simulink model "DC_motor_Fuzzy_pid_V3"  (R2020a)
settings: Solver=FixedStepAuto  StartTime=0.0  StopTime=7.5  FixedStep=0.001  RelTol=1e-3
undefined symbols (not defined in the file): sigbuilder_block
libraries: fuzblock x1
settings Model: Creator=kesha  LastModifiedBy=OMEN
settings DataIOCC: ReturnWorkspaceOutputs=off
settings DebuggingCC: ArithmeticOperatorsInVariantConditions=warning
settings SFSimCC: SimUseLocalCustomCode=off  CustomCodeUndefinedFunction=UseInterfaceOnly
settings RTWCC: RTWUseLocalCustomCode=off

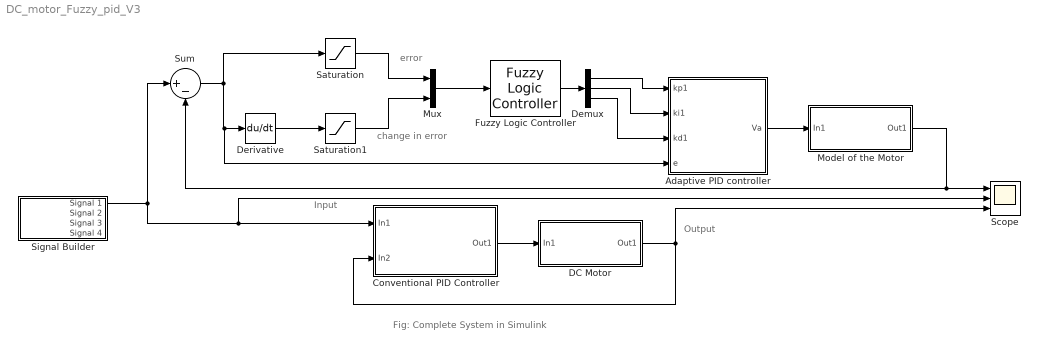
== system DC_motor_Fuzzy_pid_V3 ==
  note: change in error
  note: error
  note: Output
  note: Input
  note: Fig: Complete System in Simulink
  " Adaptive PID controller" : Subsystem  mask{Kp1=0.9989, Ki1=13.57, Kd1=0.01035}
      mask prompts: Kp1 "P"; Ki1 "I"; Kd1 "D"
      mask DialogControl ParameterGroupVar Prompt: Preliminary PID Gains
  Conventional PID Controller : Subsystem  mask{Kp=0.1, Ki=10, Kd=0.01}
      mask prompts: Kp "P"; Ki "I"; Kd "D"
  DC Motor : Subsystem
  Demux : Demux  Outputs=3
  Derivative : Derivative
  Fuzzy Logic Controller : fuzblock/Fuzzy Logic  Controller  FIS='fuzzypid.fis'  OutputSampleNumber=101  DataType=double  FuzzifiedInputs=off  RuleFiringStrengths=off  RuleOutputs=off  AggregatedOutputs=off  SimulateUsing=Interpreted execution  OutOfRangeInputValueMessage=warning  NoRuleFiredMessage=warning  EmptyOutputFuzzySetMessage=warning
  Model of the Motor : Subsystem
  Mux : Mux  Inputs=2
  Saturation : Saturate  UpperLimit=1  LowerLimit=-1  LinearizeAsGain=off  ZeroCross=off
  Saturation1 : Saturate  UpperLimit=1  LowerLimit=-1  LinearizeAsGain=off
  Scope : Scope  NumInputPorts=3
  Signal Builder : Subsystem  Tag=STV Subsys  LoadFcn=sigbuilder_block('load');  StartFcn=sigbuilder_block('start');  StopFcn=sigbuilder_block('stop');  ClipboardFcn=sigbuilder_block('clipboard');  mask(Sigbuilder block){tuvar=[0:10]}
      mask help: Simulink:masks:SigbuilderBlock_MD
      mask init:
      | if ~strcmp(get_param(bdroot(gcbh),'SimulationStatus'),'stopped') tuvar = sigbuilder_block('maskInit'); end
      settings: CopyFcn=sigbuilder_block('copy');  DeleteFcn=sigbuilder_block('delete');  ModelCloseFcn=sigbuilder_block('modelClose');  PreSaveFcn=sigbuilder_block('preSave');  PauseFcn=sigbuilder_block('pause');  ContinueFcn=sigbuilder_block('continue');  NameChangeFcn=sigbuilder_block('namechange');  OpenFcn=sigbuilder_block('open',[148.8 141 550.8 400.2 ]);  CloseFcn=sigbuilder_block('close');
      mask Display: plot(0, 0, 100, 100,[2, 2, 32, 32, 2], [68, 8, 8, 68, 68],[32, 2], [38, 38], [32, 19, 2],[53, 60, 44], [32, 17, 17, 2],[16, 16, 31, 31]);txt = getActiveGroup(gcbh);text(2, 100, txt,'verticalAlignment', 'top');
  Sum : Sum  Inputs=|+-
  wires:
  Model of the Motor/1(Out1) -> Scope/1, Sum/2
  " Adaptive PID controller"/1(Va) -> Model of the Motor/1(In1)
  Sum/1 -> Saturation/1, " Adaptive PID controller"/4(e), Derivative/1
  Derivative/1 -> Saturation1/1
  Saturation/1 -> Mux/1
  Saturation1/1 -> Mux/2
  Fuzzy Logic Controller/1 -> Demux/1
  Demux/1 -> " Adaptive PID controller"/1(kp1)
  Demux/2 -> " Adaptive PID controller"/2(ki1)
  Demux/3 -> " Adaptive PID controller"/3("kd1 ")
  Signal Builder/1(Signal 1) -> Scope/2, Conventional PID Controller/1(In1), Sum/1
  DC Motor/1(Out1) -> Scope/3, Conventional PID Controller/2(In2)
  Mux/1 -> Fuzzy Logic Controller/1
  Conventional PID Controller/1(Out1) -> DC Motor/1(In1)

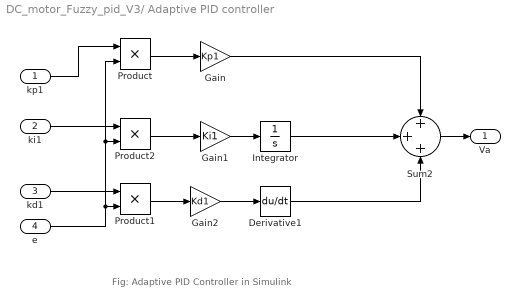
== system DC_motor_Fuzzy_pid_V3/ Adaptive PID controller ==
  note: Fig: Adaptive PID Controller in Simulink
  kp1 : Inport
  ki1 : Inport  Port=2
  "kd1 " : Inport  Port=3
  e : Inport  Port=4
  Derivative1 : Derivative
  Gain : Gain  Gain=Kp1
  Gain1 : Gain  Gain=Ki1
  Gain2 : Gain  Gain=Kd1
  Integrator : Integrator
  Product : Product
  Product1 : Product
  Product2 : Product
  Sum2 : Sum  Inputs=+++
  Va : Outport  VectorParamsAs1DForOutWhenUnconnected=off
  wires:
  Gain2/1 -> Derivative1/1
  Gain1/1 -> Integrator/1
  Sum2/1 -> Va/1
  kp1/1 -> Product/1
  ki1/1 -> Product2/1
  "kd1 "/1 -> Product1/1
  e/1 -> Product/2, Product2/2, Product1/2
  Gain/1 -> Sum2/1
  Integrator/1 -> Sum2/2
  Derivative1/1 -> Sum2/3
  Product/1 -> Gain/1
  Product2/1 -> Gain1/1
  Product1/1 -> Gain2/1

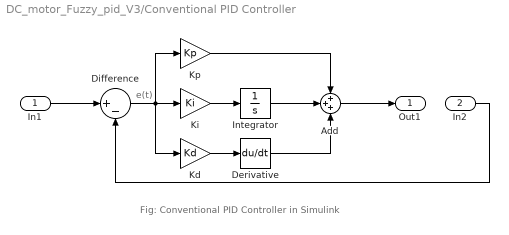
== system DC_motor_Fuzzy_pid_V3/Conventional PID Controller ==
  note: e(t)
  note: Fig: Conventional PID Controller in Simulink
  In1 : Inport
  In2 : Inport  Port=2
  " Derivative" : Derivative
  Add : Sum  Inputs=+++
  Difference : Sum  Inputs=|+-
  Integrator : Integrator
  Kd : Gain  Gain=Kd
  Ki : Gain  Gain=Ki
  Kp : Gain  Gain=Kp
  Out1 : Outport  VectorParamsAs1DForOutWhenUnconnected=off
  wires:
  " Derivative"/1 -> Add/3
  Ki/1 -> Integrator/1
  In2/1 -> Difference/2
  Integrator/1 -> Add/2
  Add/1 -> Out1/1
  In1/1 -> Difference/1
  Difference/1 -> Kd/1, Ki/1, Kp/1
  Kp/1 -> Add/1
  Kd/1 -> " Derivative"/1

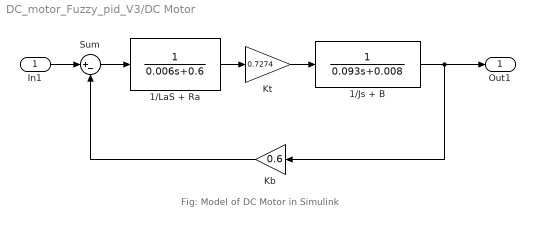
== system DC_motor_Fuzzy_pid_V3/DC Motor ==
  note: Fig: Model of DC Motor in Simulink
  In1 : Inport
  1/Js + B : TransferFcn  Denominator=[0.093 0.008]
  1/LaS + Ra : TransferFcn  Denominator=[0.006 0.6]
  Kb : Gain  Gain=0.6
  Kt : Gain  Gain=0.7274
  Sum : Sum  Inputs=|+-
  Out1 : Outport  VectorParamsAs1DForOutWhenUnconnected=off
  wires:
  1/LaS + Ra/1 -> Kt/1
  1/Js + B/1 -> Out1/1, Kb/1
  Kt/1 -> 1/Js + B/1
  Kb/1 -> Sum/2
  In1/1 -> Sum/1
  Sum/1 -> 1/LaS + Ra/1

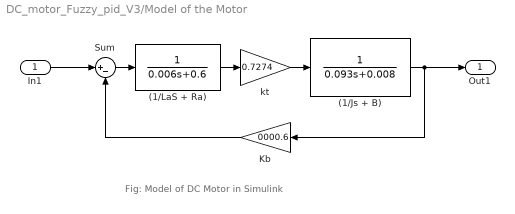
== system DC_motor_Fuzzy_pid_V3/Model of the Motor ==
  note: Fig: Model of DC Motor in Simulink
  In1 : Inport
  (1/Js + B) : TransferFcn  Denominator=[0.093 0.008]
  (1/LaS + Ra) : TransferFcn  Denominator=[0.006 0.6]
  Kb : Gain  Gain=0000.6
  Sum : Sum  Inputs=|+-
  kt : Gain  Gain=0.7274
  Out1 : Outport  VectorParamsAs1DForOutWhenUnconnected=off
  wires:
  In1/1 -> Sum/1
  Sum/1 -> (1/LaS + Ra)/1
  Kb/1 -> Sum/2
  kt/1 -> (1/Js + B)/1
  (1/Js + B)/1 -> Out1/1, Kb/1
  (1/LaS + Ra)/1 -> kt/1

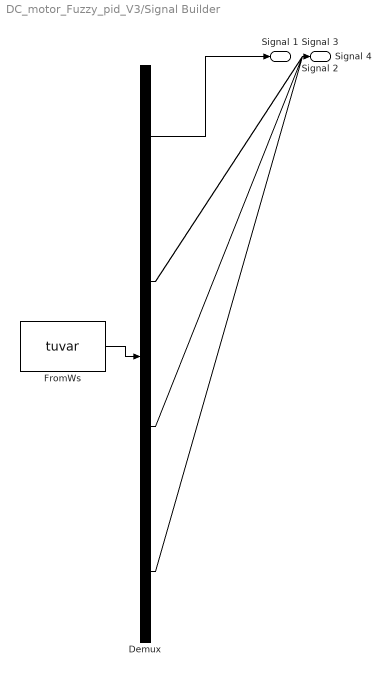
== system DC_motor_Fuzzy_pid_V3/Signal Builder ==
  Demux : Demux  Tag=STV Demux
      settings: DisplayOption=none
  FromWs : FromWorkspace  Tag=STV FromWs  VariableName=tuvar
      SigBuilderData=|
      | common.afterFinalStr = 'Extrapolate'
      | common.sampleTime = 0
      | dataSet.timeRange = [0 10]
      | dataSet.name = 'Group 1'
      | sbobj.Groups.Name = 'Group 1'
      | sbobj.Groups.Signals(1).Name = 'Signal 1'
      | sbobj.Groups.Signals(1).XData = [0 0.5 0.5 2.02 2.02 3.92 3.92 4 4 6 6 10]
      | sbobj.Groups.Signals(1).YData = [0 0 1 1 2 2 1.1 2 2.01 2.01 0.51 0.51]
      | sbobj.Groups.Signals(2).Name = 'Signal 2'
      | sbobj.Groups.Signals(2).XData = [0 0.000500500500501 0.001001001001 0.0015015015015 0.002002002002 0.0025025025025 0.003003003003 0.0035035035035 0.004004004004 0.0045045045045 0.00500500500501 0.00550550550551 ... (19981 elements, 1x19981)]
      | sbobj.Groups.Signals(2).YData = [1 1.00628943332 1.01257861784 1.01886730478 1.02515524539 1.03144219092 1.03772789268 1.04401210202 1.05029457036 1.05657504918 1.06285329004 1.06912904459 ... (19981 elements, 1x19981)]
      | sbobj.Groups.Signals(3).Name = 'Signal 3'
      | sbobj.Groups.Signals(3).XData = [0 1 1 10]
      | sbobj.Groups.Signals(3).YData = [0 0 1 1]
      | sbobj.Groups.Signals(4).Name = 'Signal 4'
      | sbobj.Groups.Signals(4).XData = [0 1 1 2 2 3 3 4 4 5 5 6 6 7 7 8 8 9 9 10]
      | sbobj.Groups.Signals(4).YData = [0 2 0 2 0 2 0 2 0 2 0 2 0 2 0 2 0 2 0 2]
  Signal 1 : Outport  Tag=STV Outport  VectorParamsAs1DForOutWhenUnconnected=off
  Signal 2 : Outport  Tag=STV Outport  Port=2  VectorParamsAs1DForOutWhenUnconnected=off
  Signal 3 : Outport  Tag=STV Outport  Port=3  VectorParamsAs1DForOutWhenUnconnected=off
  Signal 4 : Outport  Tag=STV Outport  Port=4  VectorParamsAs1DForOutWhenUnconnected=off
  wires:
  Demux/1 -> Signal 1/1
  FromWs/1 -> Demux/1
  Demux/2 -> Signal 2/1
  Demux/3 -> Signal 3/1
  Demux/4 -> Signal 4/1
